simulink model "bandwidth_velocity"  (R2020b)
settings: Solver=ode4  StartTime=0.0  StopTime=10  FixedStep=1e-5  MaxStep=1e-4  RelTol=1e-4  EnableMultiTasking=on
values from neighbouring files (symbols this model uses):
  dm = 0.0068    [bandwidth.m]    (also in bandwidth_reference.m; frequency_max_modulation_force.m; frequency_max_modulation_force_sea.m; frequency_max_modulation_position.m)
  gear = 103    [bandwidth_reference.m]    (also in frequency_max_position.m; frequency_max_velocity.m; frequency_position.m; frequency_velocity.m)
  I = 0.1    [bandwidth.m]    (also in bandwidth_reference.m = 0.2; frequency_max_modulation_velocity.m = 2; frequency_max_position.m = 0; frequency_max_velocity.m = 2)
  Jm = 0.0064    [bandwidth.m]    (also in bandwidth_reference.m = 0.0104; frequency_max_modulation_force.m = 0.0104; frequency_max_modulation_force_sea.m = 0.0104; frequency_max_modulation_position.m = 0.0104)
  kt = 1.5038    [bandwidth_reference.m]    (also in frequency_max_modulation_force.m; frequency_max_modulation_force_sea.m; frequency_max_modulation_position.m; frequency_max_modulation_velocity.m)
  P = 15    [bandwidth.m]    (also in bandwidth_reference.m = 1; frequency_max_modulation_force.m = 10; frequency_max_modulation_force_sea.m = 10; frequency_max_modulation_position.m = 10)
  R = 0.68    [bandwidth_reference.m]
settings Model: Creator=eldisondimo  LastModifiedBy=filippo
settings DataIOCC: LimitDataPoints=on  SaveOutput=off  SaveTime=off  ReturnWorkspaceOutputs=off
settings OptimizationCC: ExpressionDepthLimit=2147483647  LifeSpan=1
settings DebuggingCC: UnderspecifiedInitializationDetection=Classic  MergeDetectMultiDrivingBlocksExec=none  FcnCallInpInsideContextMsg=warning  AllowSymbolicDim=off  StateNameClashWarn=warning  SFUnexpectedBacktrackingDiag=warning  SFNoUnconditionalDefaultTransitionDiag=warning  SFExecutionAtInitializationDiag=none  ArithmeticOperatorsInVariantConditions=warning
settings SFSimCC: SimUseLocalCustomCode=off  CustomCodeUndefinedFunction=UseInterfaceOnly
settings RTWCC: RTWUseLocalCustomCode=off
settings CodeAppCC: StateflowObjectComments=on
settings GRTTargetCC: TargetLangStandard=C89/C90 (ANSI)  CombineOutputUpdateFcns=off  GRTInterface=on

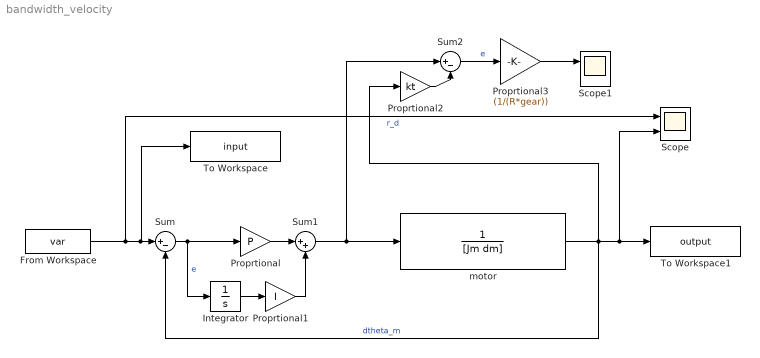
== system bandwidth_velocity ==
  From Workspace : FromWorkspace  VariableName=var
  Integrator : Integrator
  Proprtional : Gain  Gain=P
  Proprtional1 : Gain  Gain=I
  Proprtional2 : Gain  Gain=kt
  Proprtional3 : Gain  Gain=(1/(R*gear))
  Scope : Scope  NumInputPorts=2
  Scope1 : Scope  NumInputPorts=2
  Sum : Sum  Inputs=|+-
  Sum1 : Sum  Inputs=|++
  Sum2 : Sum  Inputs=|+-
  To Workspace : ToWorkspace  VariableName=input  SaveFormat=Structure With Time  SampleTime=-1
  To Workspace1 : ToWorkspace  VariableName=output  SaveFormat=Structure With Time  SampleTime=-1
  "motor " : TransferFcn  Denominator=[Jm dm]
  wires:
  From Workspace/1 -> Scope/1, To Workspace/1, Sum/1  "r_d"
  "motor "/1 -> Proprtional2/1, To Workspace1/1, Scope/2, Sum/2  "dtheta_m"
  Proprtional/1 -> Sum1/1
  Integrator/1 -> Proprtional1/1
  Sum/1 -> Integrator/1, Proprtional/1  "e"
  Sum1/1 -> Sum2/1, "motor "/1
  Proprtional1/1 -> Sum1/2
  Proprtional2/1 -> Sum2/2
  Sum2/1 -> Proprtional3/1  "e"
  Proprtional3/1 -> Scope1/1
